simulink model "esercitazione1"  (R2023b)
settings: Solver=VariableStepAuto  StartTime=0.0  StopTime=12000  MaxStep=0.01  RelTol=1e-3
InitFcn:
  | init
values from neighbouring files (symbols this model uses):
  A_Fx = 2e-8    (= 2e-08)    [init.m]
  A_Fy = 1e-8    (= 1e-08)    [init.m]
  A_Fz = 4e-8    (= 4e-08)    [init.m]
  f_Fx = 5e-3    (= 0.005)    [init.m]
  f_Fy = 9e-3    (= 0.009)    [init.m]
  f_Fz = 2e-2    (= 0.02)    [init.m]
  I = [I_x; I_y; I_z]    [init.m]
  ph_Fx = pi/2    (= 1.57079632679)    [init.m]
  ph_Fy = pi/2    (= 1.57079632679)    [init.m]
  ph_Fz = pi/2    (= 1.57079632679)    [init.m]
  qi = [1; 0; 0; 0]    [init.m]
  w_ic = [0; -w_o; 0]    [init.m]
libraries: sharedtransform x1
settings Model: Creator=dario  LastModifiedBy=dario

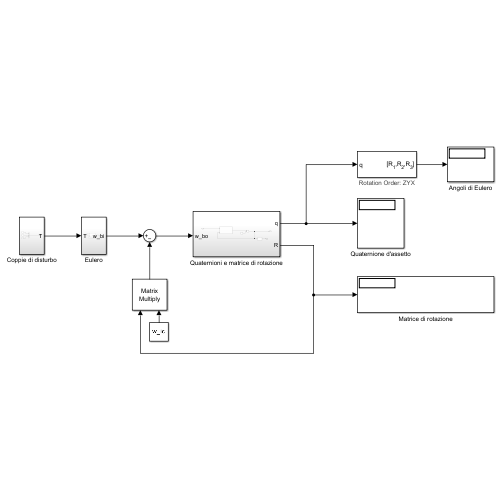
[thumbnail: Simulink's stored preview of the top-level diagram]
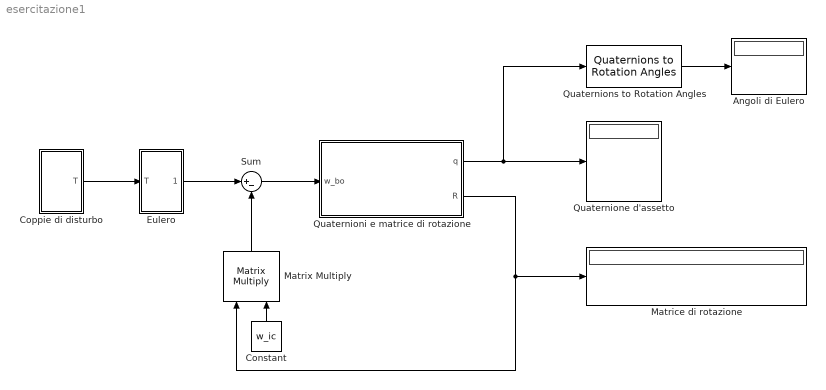
== system esercitazione1 ==
  Angoli di Eulero : Display
  Constant : Constant  Value=w_ic  VectorParams1D=off
  Coppie di disturbo : Subsystem
  Eulero : Subsystem
  Matrice di rotazione : Display
  Matrix Multiply : Product  Inputs=**  Multiplication=Matrix(*)
  Quaternione d'assetto : Display
  Quaternioni e matrice di rotazione : Subsystem
  Quaternions to Rotation Angles : sharedtransform/Quaternions to Rotation Angles  rotationOrder=ZYX  aMode=aMode
  Sum : Sum  Inputs=|+-
  wires:
  Constant/1 -> Matrix Multiply/2
  Matrix Multiply/1 -> Sum/2
  Coppie di disturbo/1(T) -> Eulero/1(T)
  Eulero/1(w_bi) -> Sum/1
  Quaternioni e matrice di rotazione/2(R) -> Matrix Multiply/1, Matrice di rotazione/1
  Sum/1 -> Quaternioni e matrice di rotazione/1(w_bo)
  Quaternioni e matrice di rotazione/1(q) -> Quaternions to Rotation Angles/1, Quaternione d'assetto/1
  Quaternions to Rotation Angles/1 -> Angoli di Eulero/1

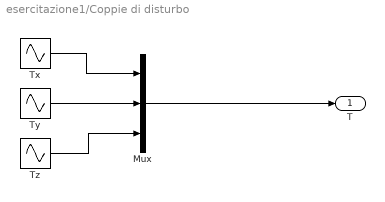
== system esercitazione1/Coppie di disturbo ==
  Mux : Mux  Inputs=3
  Tx : Sin  Amplitude=A_Fx  Frequency=f_Fx  Phase=ph_Fx  SampleTime=0
  Ty : Sin  Amplitude=A_Fy  Frequency=f_Fy  Phase=ph_Fy  SampleTime=0
  Tz : Sin  Amplitude=A_Fz  Frequency=f_Fz  Phase=ph_Fz  SampleTime=0
  T : Outport
  wires:
  Ty/1 -> Mux/2
  Tz/1 -> Mux/3
  Tx/1 -> Mux/1
  Mux/1 -> T/1

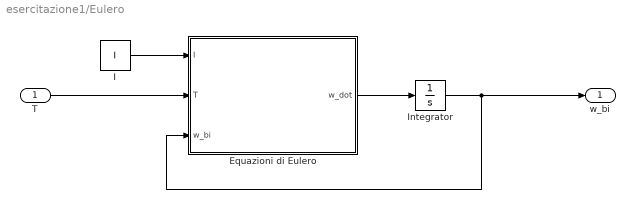
== system esercitazione1/Eulero ==
  T : Inport
  Equazioni di Eulero : MATLAB Function  TreatAsAtomicUnit=on
  I : Constant  Value=I  VectorParams1D=off
  Integrator : Integrator  InitialCondition=w_ic
  w_bi : Outport
  wires:
  I/1 -> Equazioni di Eulero/1(I)
  Equazioni di Eulero/1(w_dot) -> Integrator/1
  Integrator/1 -> w_bi/1, Equazioni di Eulero/3(w_bi)
  T/1 -> Equazioni di Eulero/2(T)

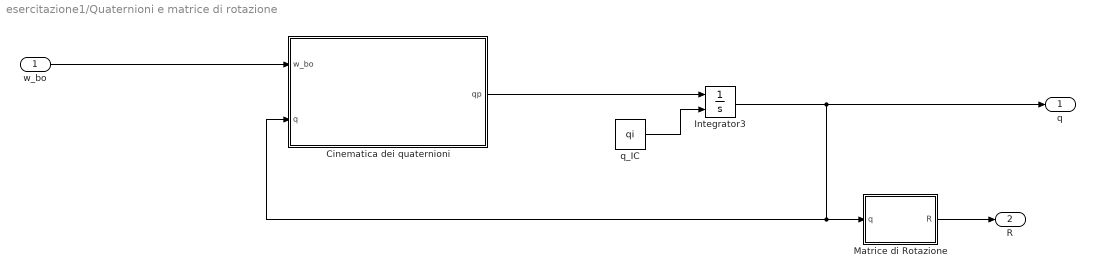
== system esercitazione1/Quaternioni e matrice di rotazione ==
  w_bo : Inport
  Cinematica dei quaternioni : MATLAB Function  TreatAsAtomicUnit=on
  Integrator3 : Integrator  InitialConditionSource=external
  Matrice di Rotazione : MATLAB Function  TreatAsAtomicUnit=on
  q_IC : Constant  Value=qi  VectorParams1D=off
  q : Outport
  R : Outport  Port=2
  wires:
  Integrator3/1 -> q/1, Cinematica dei quaternioni/2(q), Matrice di Rotazione/1(q)
  q_IC/1 -> Integrator3/2
  Matrice di Rotazione/1(R) -> R/1
  Cinematica dei quaternioni/1(qp) -> Integrator3/1
  w_bo/1 -> Cinematica dei quaternioni/1(w_bo)

== matlab function esercitazione1/Quaternioni e matrice di rotazione/Cinematica dei quaternioni ==
  data: w_bo input; qp output; q input
function qp = Quaternioni(w_bo,q)
w_box=w_bo(1);
w_boy=w_bo(2);
w_boz=w_bo(3);

Q=[0 -w_box -w_boy -w_boz;
    w_box 0 w_boz -w_boy; 
    w_boy -w_boz 0 w_box; 
    w_boz w_boy -w_box 0];

qp=0.5*Q*q;

== matlab function esercitazione1/Eulero/Equazioni di Eulero ==
  data: I input; w_dot output; T input; w_bi input
function w_dot = Eulero(I,T,w_bi)
I_x=I(1);
I_y=I(2);
I_z=I(3);
T_x=T(1);
T_y=T(2);
T_z=T(3);
w_bix=w_bi(1);
w_biy=w_bi(2);
w_biz=w_bi(3);
a_x=-w_biy*w_biz*((I_z-I_y)/(I_x))+T_x/I_x;
a_y=-w_bix*w_biz*((I_x-I_z)/(I_y))+T_y/I_y;
a_z=-w_bix*w_biy*((I_y-I_x)/(I_z))+T_z/I_z;

w_dot=[a_x;a_y;a_z];

== matlab function esercitazione1/Quaternioni e matrice di rotazione/Matrice di Rotazione ==
  data: q input; R output
function R = rotmat(q)
i=eye(3);
qdir=[q(2); q(3); q(4)];
A=[0 -q(4) q(3); q(4) 0 -q(2); -q(3) q(2) 0];
R=(q(1)^2-dot(qdir,qdir))*i+2*(qdir*qdir')-2*q(1)*A;
